simulink model "linear_acceleration"  (R2024b)
settings: Solver=VariableStepAuto  StartTime=0.0  StopTime=10.0  RelTol=1e-3
settings Model: Creator=shohei  LastModifiedBy=shohei

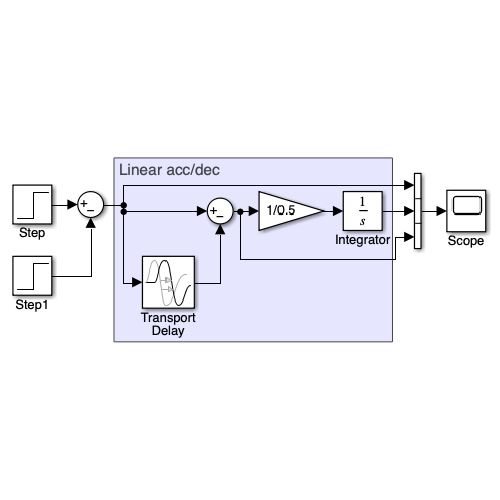
[thumbnail: Simulink's stored preview of the top-level diagram]
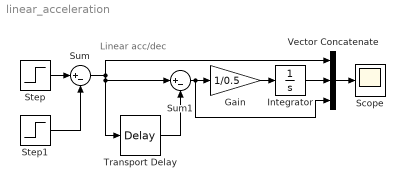
== system linear_acceleration ==
  note: Linear acc/dec
  Gain : Gain  Gain=1/0.5
  Integrator : Integrator
  Scope : Scope
  Step : Step  SampleTime=0
  Step1 : Step  Time=5  SampleTime=0
  Sum : Sum  Inputs=|+-
  Sum1 : Sum  Inputs=|+-
  Transport Delay : TransportDelay  DelayTime=0.5
  Vector Concatenate : Concatenate  NumInputs=3
  wires:
  Gain/1 -> Integrator/1
  Sum/1 -> Transport Delay/1, Sum1/1, Vector Concatenate/1
  Step1/1 -> Sum/2
  Step/1 -> Sum/1
  Vector Concatenate/1 -> Scope/1
  Sum1/1 -> Vector Concatenate/3, Gain/1
  Integrator/1 -> Vector Concatenate/2
  Transport Delay/1 -> Sum1/2
